simulink model "lpf"  (Simulink 7.7)
settings: Solver=ode4  StartTime=0.0  StopTime=10.0  FixedStep=0.00434  RelTol=1e-3
settings Model: Creator=Fede  LastModifiedBy=Fede
settings OptimizationCC: OptimizeModelRefInitCode=on  LifeSpan=1
settings RTWCC: SystemTargetFile=ert.tlc  GenCodeOnly=on  TemplateMakefile=ert_default_tmf  Description=Embedded Coder  ProcessScript=ert_make_rtw_hook  RTWCompilerOptimization=On
settings CodeAppCC: IgnoreCustomStorageClasses=off
settings ERTTargetCC: FunctionExecutionProfile=off  MultiwordLength=2048  GenerateSampleERTMain=on  ERTCustomFileTemplate=example_file_process.tlc  ConvertIfToSwitch=off

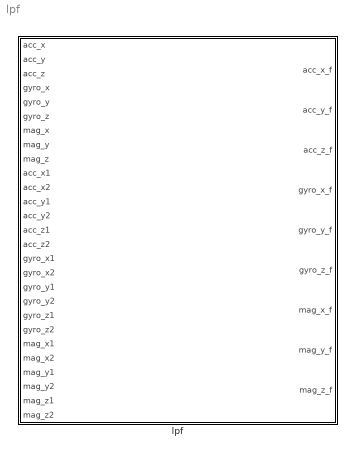
== system lpf ==
  lpf : Subsystem

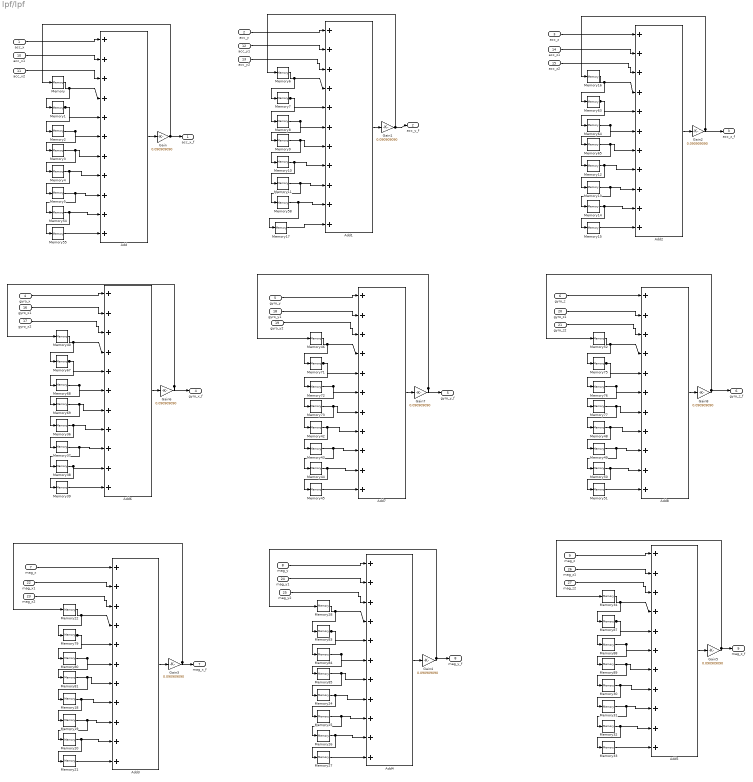
== system lpf/lpf ==
  acc_x : Inport  OutMin=-20  OutMax=20  OutDataTypeStr=double
  acc_y : Inport  Port=2  OutMin=-20  OutMax=20  OutDataTypeStr=double
  acc_z : Inport  Port=3  OutMin=-20  OutMax=20  OutDataTypeStr=double
  gyro_x : Inport  Port=4  OutDataTypeStr=double
  gyro_y : Inport  Port=5  OutDataTypeStr=double
  gyro_z : Inport  Port=6  OutDataTypeStr=double
  mag_x : Inport  Port=7  OutDataTypeStr=double
  mag_y : Inport  Port=8  OutDataTypeStr=double
  mag_z : Inport  Port=9  OutDataTypeStr=double
  acc_x1 : Inport  Port=10  OutMin=-20  OutMax=20  OutDataTypeStr=double
  acc_x2 : Inport  Port=11  OutMin=-20  OutMax=20  OutDataTypeStr=double
  acc_y1 : Inport  Port=12  OutMin=-20  OutMax=20  OutDataTypeStr=double
  acc_y2 : Inport  Port=13  OutMin=-20  OutMax=20  OutDataTypeStr=double
  acc_z1 : Inport  Port=14  OutMin=-20  OutMax=20  OutDataTypeStr=double
  acc_z2 : Inport  Port=15  OutMin=-20  OutMax=20  OutDataTypeStr=double
  gyro_x1 : Inport  Port=16  OutDataTypeStr=double
  gyro_x2 : Inport  Port=17  OutDataTypeStr=double
  gyro_y1 : Inport  Port=18  OutDataTypeStr=double
  gyro_y2 : Inport  Port=19  OutDataTypeStr=double
  gyro_z1 : Inport  Port=20  OutDataTypeStr=double
  gyro_z2 : Inport  Port=21  OutDataTypeStr=double
  mag_x1 : Inport  Port=22  OutDataTypeStr=double
  mag_x2 : Inport  Port=23  OutDataTypeStr=double
  mag_y1 : Inport  Port=24  OutDataTypeStr=double
  mag_y2 : Inport  Port=25  OutDataTypeStr=double
  mag_z1 : Inport  Port=26  OutDataTypeStr=double
  mag_z2 : Inport  Port=27  OutDataTypeStr=double
  Add{,1..8} (9 alike) : Sum  Inputs=+++++++++++  AccumDataTypeStr=double  OutMin=-20  OutMax=20  OutDataTypeStr=single  SampleTime=0.00434
  Gain{,1..8} (9 alike) : Gain  Gain=0.090909090  OutDataTypeStr=double  SampleTime=0.00434
  Memory{,1..22,24..28,30..34,36..40,42..46,48..52,54..55,58,63..65,67..69,71..73,75..77,79..81,83..85,87..89} (72 alike) : Memory
  acc_x_f : Outport  OutDataTypeStr=double
  acc_y_f : Outport  Port=2  OutDataTypeStr=double
  acc_z_f : Outport  Port=3  OutDataTypeStr=double
  gyro_x_f : Outport  Port=4  OutDataTypeStr=double
  gyro_y_f : Outport  Port=5  OutDataTypeStr=double
  gyro_z_f : Outport  Port=6  OutDataTypeStr=double
  mag_x_f : Outport  Port=7  OutDataTypeStr=double
  mag_y_f : Outport  Port=8  OutDataTypeStr=double
  mag_z_f : Outport  Port=9  OutDataTypeStr=double
  wires:
  Memory/1 -> Memory1/1, Add/4
  Add/1 -> Gain/1
  Memory1/1 -> Memory2/1, Add/5
  Memory2/1 -> Memory3/1, Add/6
  Memory3/1 -> Memory4/1, Add/7
  Memory4/1 -> Memory5/1, Add/8
  Gain/1 -> Memory/1, acc_x_f/1
  acc_x/1 -> Add/1
  acc_x1/1 -> Add/2
  acc_x2/1 -> Add/3
  Memory5/1 -> Add/9, Memory54/1
  Memory54/1 -> Add/10, Memory55/1
  Memory55/1 -> Add/11
  Memory6/1 -> Add1/4, Memory7/1
  Add1/1 -> Gain1/1
  Memory7/1 -> Add1/5, Memory8/1
  Memory8/1 -> Add1/6, Memory9/1
  Memory9/1 -> Add1/7, Memory10/1
  Memory10/1 -> Add1/8, Memory11/1
  Gain1/1 -> Memory6/1, acc_y_f/1
  acc_y/1 -> Add1/1
  acc_y1/1 -> Add1/2
  acc_y2/1 -> Add1/3
  Memory11/1 -> Memory58/1, Add1/9
  Memory58/1 -> Add1/10, Memory17/1
  Memory16/1 -> Add2/4, Memory63/1
  Add2/1 -> Gain2/1
  Memory63/1 -> Add2/5, Memory64/1
  Memory64/1 -> Add2/6, Memory65/1
  Memory65/1 -> Add2/7, Memory12/1
  Memory12/1 -> Add2/8, Memory13/1
  Gain2/1 -> Memory16/1, acc_z_f/1
  acc_z/1 -> Add2/1
  acc_z1/1 -> Add2/2
  acc_z2/1 -> Add2/3
  Memory13/1 -> Memory14/1, Add2/9
  Memory14/1 -> Memory15/1, Add2/10
  Memory15/1 -> Add2/11
  Memory40/1 -> Add6/4, Memory67/1
  Add6/1 -> Gain6/1
  Memory67/1 -> Add6/5, Memory68/1
  Memory68/1 -> Add6/6, Memory69/1
  Memory69/1 -> Add6/7, Memory36/1
  Memory36/1 -> Add6/8, Memory37/1
  Gain6/1 -> Memory40/1, gyro_x_f/1
  gyro_x/1 -> Add6/1
  gyro_x1/1 -> Add6/2
  gyro_x2/1 -> Add6/3
  Memory37/1 -> Memory38/1, Add6/9
  Memory38/1 -> Memory39/1, Add6/10
  Memory46/1 -> Add7/4, Memory71/1
  Add7/1 -> Gain7/1
  Memory71/1 -> Add7/5, Memory72/1
  Memory72/1 -> Add7/6, Memory73/1
  Memory73/1 -> Add7/7, Memory42/1
  Memory42/1 -> Add7/8, Memory43/1
  Gain7/1 -> Memory46/1, gyro_y_f/1
  gyro_y/1 -> Add7/1
  gyro_y1/1 -> Add7/2
  gyro_y2/1 -> Add7/3
  Memory43/1 -> Memory44/1, Add7/9
  Memory44/1 -> Memory45/1, Add7/10
  Memory45/1 -> Add7/11
  Memory52/1 -> Add8/4, Memory75/1
  Add8/1 -> Gain8/1
  Memory75/1 -> Add8/5, Memory76/1
  Memory76/1 -> Add8/6, Memory77/1
  Memory77/1 -> Add8/7, Memory48/1
  Memory48/1 -> Add8/8, Memory49/1
  Gain8/1 -> Memory52/1, gyro_z_f/1
  gyro_z/1 -> Add8/1
  gyro_z1/1 -> Add8/2
  gyro_z2/1 -> Add8/3
  Memory49/1 -> Memory50/1, Add8/9
  Memory50/1 -> Memory51/1, Add8/10
  Memory51/1 -> Add8/11
  Memory22/1 -> Add3/4, Memory79/1
  Add3/1 -> Gain3/1
  Memory79/1 -> Add3/5, Memory80/1
  Memory80/1 -> Add3/6, Memory81/1
  Memory81/1 -> Add3/7, Memory18/1
  Memory18/1 -> Add3/8, Memory19/1
  Gain3/1 -> Memory22/1, mag_x_f/1
  mag_x/1 -> Add3/1
  mag_x1/1 -> Add3/2
  mag_x2/1 -> Add3/3
  Memory19/1 -> Memory20/1, Add3/9
  Memory20/1 -> Memory21/1, Add3/10
  Memory21/1 -> Add3/11
  Memory28/1 -> Add4/4, Memory83/1
  Add4/1 -> Gain4/1
  Memory83/1 -> Add4/5, Memory84/1
  Memory84/1 -> Add4/6, Memory85/1
  Memory85/1 -> Add4/7, Memory24/1
  Memory24/1 -> Add4/8, Memory25/1
  Gain4/1 -> Memory28/1, mag_y_f/1
  mag_y/1 -> Add4/1
  mag_y1/1 -> Add4/2
  mag_y2/1 -> Add4/3
  Memory25/1 -> Memory26/1, Add4/9
  Memory26/1 -> Memory27/1, Add4/10
  Memory27/1 -> Add4/11
  Memory34/1 -> Add5/4, Memory87/1
  Add5/1 -> Gain5/1
  Memory87/1 -> Add5/5, Memory88/1
  Memory88/1 -> Add5/6, Memory89/1
  Memory89/1 -> Add5/7, Memory30/1
  Memory30/1 -> Add5/8, Memory31/1
  Gain5/1 -> Memory34/1, mag_z_f/1
  mag_z/1 -> Add5/1
  mag_z1/1 -> Add5/2
  mag_z2/1 -> Add5/3
  Memory31/1 -> Memory32/1, Add5/9
  Memory32/1 -> Memory33/1, Add5/10
  Memory33/1 -> Add5/11
  Memory17/1 -> Add1/11
  Memory39/1 -> Add6/11
